simulink model "site_grid_behavior_ev_charging"  (R2025b)
settings: Solver=ode3  StartTime=0.0  StopTime=86400  FixedStep=300  RelTol=1e-3
settings Model: Creator=adand  LastModifiedBy=adand

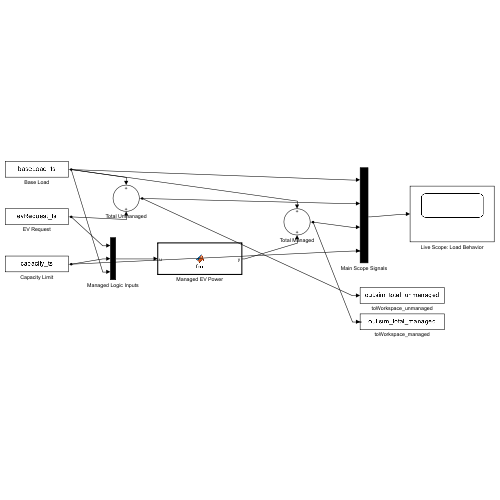
[thumbnail: Simulink's stored preview of the top-level diagram]
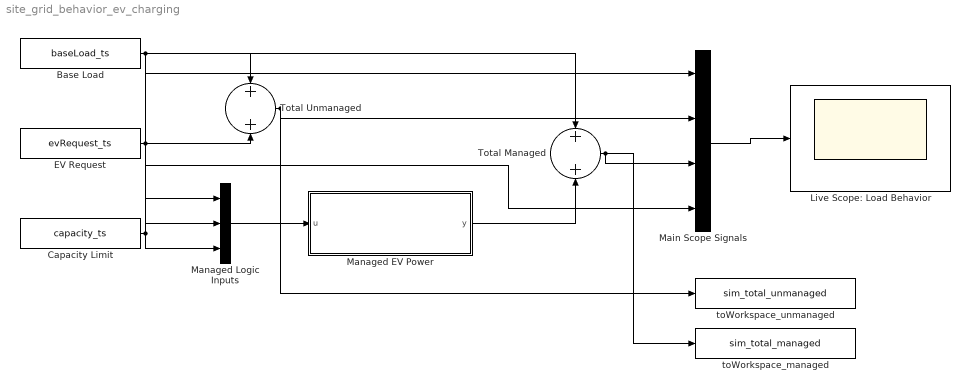
== system site_grid_behavior_ev_charging ==
  Base Load : FromWorkspace  VariableName=baseLoad_ts
  Capacity Limit : FromWorkspace  VariableName=capacity_ts
  EV Request : FromWorkspace  VariableName=evRequest_ts
  Live Scope: Load Behavior : Scope
  Main Scope Signals : Mux
  Managed EV Power : MATLAB Function  TreatAsAtomicUnit=on
  Managed Logic Inputs : Mux  Inputs=3
  Total Managed : Sum
  Total Unmanaged : Sum
  toWorkspace_managed : ToWorkspace  VariableName=sim_total_managed  SaveFormat=Structure With Time  SampleTime=-1
  toWorkspace_unmanaged : ToWorkspace  VariableName=sim_total_unmanaged  SaveFormat=Structure With Time  SampleTime=-1
  wires:
  Base Load/1 -> Total Unmanaged/1, Managed Logic Inputs/3, Total Managed/1, Main Scope Signals/1
  EV Request/1 -> Total Unmanaged/2, Managed Logic Inputs/1
  Capacity Limit/1 -> Managed Logic Inputs/2, Main Scope Signals/4
  Managed Logic Inputs/1 -> Managed EV Power/1(u)
  Managed EV Power/1(y) -> Total Managed/2
  Total Unmanaged/1 -> Main Scope Signals/2, toWorkspace_unmanaged/1
  Total Managed/1 -> Main Scope Signals/3, toWorkspace_managed/1
  Main Scope Signals/1 -> Live Scope: Load Behavior/1

== matlab function site_grid_behavior_ev_charging/Managed EV Power ==
  data: u input; y output
function y = fcn(u)
% u(1) = EV request
% u(2) = site capacity
% u(3) = base building load
available = max(u(2) - u(3), 0);
y = min(u(1), available);
end
